simulink model "SVMInverter"  (R2022b)
settings: Solver=ode4  StartTime=0.0  StopTime=0.06  FixedStep=1e-6  RelTol=1e-3
values from neighbouring files (symbols this model uses):
  Cf = 1/(Lf*wc^2)    (= 0.000101321183642)    [FOCinit.m]
  E = 700    [FOCinit.m]
  Lf = 1e-3    (= 0.001)    [FOCinit.m]
  Ls = 0.280    (= 0.28)    [FOCinit.m]
  Poff = [1 1 1 1 1 1 1 1 1 1 1 1 1 1 1 1 1 1 ; 1 0 0 1 1 0 0 1 0 0 1 1 0 0 1 1 0 1; 1 1 0 0 1 0 0 1 1 0 0 1 1 0 1 1 0 0]'    [FOCinit.m]
  Rf = (1/(2*eps))*sqrt(Lf/Cf)    [FOCinit.m]
  Ts = 1/fs    (= 0.0001)    [FOCinit.m]
libraries: simulink_extras x6, simulink x2, mcbcontrolslib x2
settings Model: Creator=ZinouAb  LastModifiedBy=ZinouAb

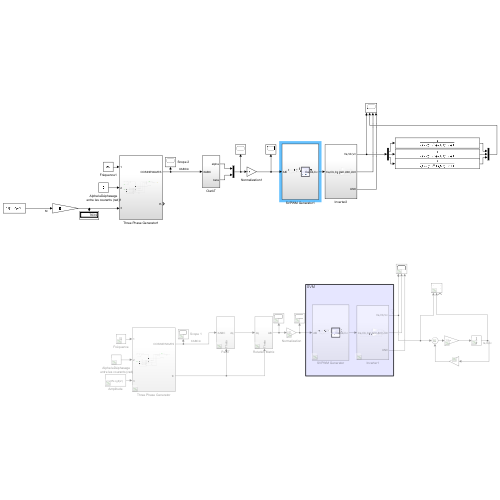
[thumbnail: Simulink's stored preview of the top-level diagram]
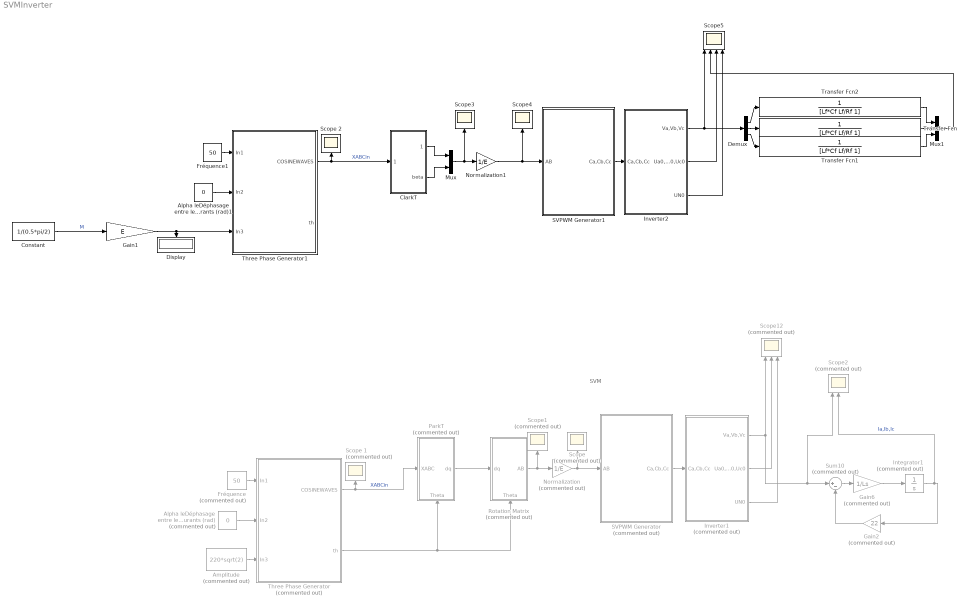
== system SVMInverter ==
  note: SVM
  Alpha leDéphasage entre les courants (rad) : Constant  Commented=on  Value=0
  Alpha leDéphasage entre les courants (rad)1 : Constant  Value=0
  Amplitude : Constant  Commented=on  Value=220*sqrt(2)
  ClarkT : Subsystem
  Constant : Constant  Value=1/(0.5*pi/2)
  Demux : Demux  Outputs=3
  Display : Display
  Fréquence : Constant  Commented=on  Value=50
  Fréquence1 : Constant  Value=50
  Gain1 : Gain  Gain=E
  Gain2 : Gain  Commented=on  Gain=22
  Gain6 : Gain  Commented=on  Gain=1/Ls
  Integrator1 : Integrator  Commented=on
  Inverter1 : Subsystem  Commented=on
  Inverter2 : Subsystem
  Mux : Mux  Inputs=2
  Mux1 : Mux  Inputs=3
  Normalization : Gain  Commented=on  Gain=1/E
  Normalization1 : Gain  Gain=1/E
  ParkT : Subsystem  Commented=on
      settings: PortSchema="{\"entries\":[{\"content\":{\"sides\":[{\"content\":{\"connectorIds\":[\"In1\"]},\"type\":\"ConnectorPlacement.EquallySpacedRectSide\",\"uuid\":\"228dfcfc-5d6b-4d2b-a954-ee5f3fee8856\"},{\"content\":{\"connectorIds\":[\"Out1\"],\"side\":\"RIGHT\"},\"type\":\"ConnectorPlacement.EquallySpacedRectSide\",\"uuid\":\"1b1b4c30-bceb-4aa5-9a3a-183aa9b64903\"},{\"content\":{\"connectorIds\":[],\"side\":\"TOP\"},\"type\":\"ConnectorPlacement.EquallySpacedRectSide\",\"uuid\":\"f7d3bddd-1df8-4cd8-ab8f-9e5cd0980ffa\"},{\"content\":{\"connectorIds\":[\"In2\"],\"side\":\"BOTTOM\"},\"type\":\"ConnectorPlacement.EquallySpacedRectSide\",\"uuid\":\"ca51e6a4-16df-4fde-8b7d-f74278a3171d\"}]},\"type\":\"ConnectorPlacement.EquallySpacedConnector\",\"uuid\":\"a8efb2f9-24b2-4419-8f97-2809a6aaa24c\"}],\"packageUris\":[\"http://schema.mathworks.com/mf0/Connector/R2020b\"],\"version\":\"1.0\"}"
  Rotation Matrix : Subsystem  Commented=on
      settings: PortSchema="{\"entries\":[{\"content\":{\"sides\":[{\"content\":{\"connectorIds\":[\"In1\"]},\"type\":\"ConnectorPlacement.EquallySpacedRectSide\",\"uuid\":\"228dfcfc-5d6b-4d2b-a954-ee5f3fee8856\"},{\"content\":{\"connectorIds\":[\"Out1\"],\"side\":\"RIGHT\"},\"type\":\"ConnectorPlacement.EquallySpacedRectSide\",\"uuid\":\"1b1b4c30-bceb-4aa5-9a3a-183aa9b64903\"},{\"content\":{\"connectorIds\":[],\"side\":\"TOP\"},\"type\":\"ConnectorPlacement.EquallySpacedRectSide\",\"uuid\":\"f7d3bddd-1df8-4cd8-ab8f-9e5cd0980ffa\"},{\"content\":{\"connectorIds\":[\"In2\"],\"side\":\"BOTTOM\"},\"type\":\"ConnectorPlacement.EquallySpacedRectSide\",\"uuid\":\"ca51e6a4-16df-4fde-8b7d-f74278a3171d\"}]},\"type\":\"ConnectorPlacement.EquallySpacedConnector\",\"uuid\":\"a8efb2f9-24b2-4419-8f97-2809a6aaa24c\"}],\"packageUris\":[\"http://schema.mathworks.com/mf0/Connector/R2020b\"],\"version\":\"1.0\"}"
  SVPWM Generator : Subsystem  Commented=on
  SVPWM Generator1 : Subsystem
  Scope : Scope  Commented=on
  Scope 1 : Scope  Commented=on
  Scope 2 : Scope
  Scope1 : Scope  Commented=on
  Scope12 : Scope  Commented=on  NumInputPorts=3
  Scope2 : Scope  Commented=on  NumInputPorts=3
  Scope3 : Scope
  Scope4 : Scope
  Scope5 : Scope  NumInputPorts=4
  Sum10 : Sum  Commented=on  Inputs=|+-
  Three Phase Generator : Subsystem  Commented=on
  Three Phase Generator1 : Subsystem
  Transfer Fcn : TransferFcn  Denominator=[Lf*Cf Lf/Rf 1]
  Transfer Fcn1 : TransferFcn  Denominator=[Lf*Cf Lf/Rf 1]
  Transfer Fcn2 : TransferFcn  Denominator=[Lf*Cf Lf/Rf 1]
  wires:
  Integrator1/1 -> Scope2/2, Gain2/1  "Ia,Ib,Ic"
  Inverter1/1(Va,Vb,Vc) -> Scope12/1, Scope2/1, Sum10/1
  Three Phase Generator/1(COSINEWAVES) -> ParkT/1(XABC), Scope 1/1  "XABCin"
  Amplitude/1 -> Three Phase Generator/3(In3)
  Alpha leDéphasage entre les courants (rad)/1 -> Three Phase Generator/2(In2)
  Fréquence/1 -> Three Phase Generator/1(In1)
  Gain2/1 -> Sum10/2
  Gain6/1 -> Integrator1/1
  Sum10/1 -> Gain6/1
  Inverter1/2(Ua0,Ub0,Uc0) -> Scope12/2
  Inverter1/3(UN0) -> Scope12/3
  Rotation Matrix/1(AB) -> Scope1/1, Normalization/1
  Normalization/1 -> SVPWM Generator/1(AB), Scope/1
  Three Phase Generator/2(th) -> ParkT/2(Theta), Rotation Matrix/2(Theta)
  ParkT/1(dq) -> Rotation Matrix/1(dq)
  SVPWM Generator/1(Ca,Cb,Cc) -> Inverter1/1(Ca,Cb,Cc)
  Three Phase Generator1/1(COSINEWAVES) -> ClarkT/1(XABC), Scope 2/1  "XABCin"
  Fréquence1/1 -> Three Phase Generator1/1(In1)
  Alpha leDéphasage entre les courants (rad)1/1 -> Three Phase Generator1/2(In2)
  ClarkT/1(alpha) -> Mux/1
  ClarkT/2(beta) -> Mux/2
  Mux/1 -> Scope3/1, Normalization1/1
  Normalization1/1 -> Scope4/1, SVPWM Generator1/1(AB)
  Inverter2/2(Ua0,Ub0,Uc0) -> Scope5/3
  Inverter2/1(Va,Vb,Vc) -> Scope5/1, Demux/1
  Inverter2/3(UN0) -> Scope5/4
  SVPWM Generator1/1(Ca,Cb,Cc) -> Inverter2/1(Ca,Cb,Cc)
  Mux1/1 -> Scope5/2
  Demux/2 -> Transfer Fcn/1
  Demux/1 -> Transfer Fcn2/1
  Demux/3 -> Transfer Fcn1/1
  Transfer Fcn/1 -> Mux1/2
  Transfer Fcn2/1 -> Mux1/1
  Transfer Fcn1/1 -> Mux1/3
  Constant/1 -> Gain1/1  "M"
  Gain1/1 -> Three Phase Generator1/3(In3), Display/1

== system SVMInverter/ClarkT ==
  XABC : Inport
  MATLAB Function1 : MATLAB Function  TreatAsAtomicUnit=on
  alpha : Outport
  beta : Outport  Port=2
  wires:
  MATLAB Function1/1(alpha) -> alpha/1
  XABC/1 -> MATLAB Function1/1(x)
  MATLAB Function1/2(beta) -> beta/1

== system SVMInverter/Inverter1 ==
  Ca,Cb,Cc : Inport
  Constant1 : Constant  Value=E
  Gain : Gain  Gain=1/3
  Gain1 : Gain  Gain=eye(3)  Multiplication=Matrix(K*u)
  Gain2 : Gain  Gain=[2 -1 -1; -1 2 -1; -1 -1 2]  Multiplication=Matrix(K*u)
  Gain6 : Gain  Gain=1/3
  Product1 : Product
  Product3 : Product
  Scope6 : Scope
  Sum of Elements : Sum  Inputs=+
  Va,Vb,Vc : Outport
  Ua0,Ub0,Uc0 : Outport  Port=2
  UN0 : Outport  Port=3
  wires:
  Gain2/1 -> Gain6/1
  Product3/1 -> Va,Vb,Vc/1  "Va,Vb,Vc"
  Ca,Cb,Cc/1 -> Gain1/1, [Cmd], Gain2/1, Scope6/1  "Ca,Cb,Cc"
  Constant1/1 -> Product1/2, Product3/2  "U0"
  Gain6/1 -> Product3/1
  Gain1/1 -> Product1/1
  Product1/1 -> Sum of Elements/1, Ua0,Ub0,Uc0/1  "Ua0,Ub0,Uc0"
  Sum of Elements/1 -> Gain/1
  Gain/1 -> UN0/1

== system SVMInverter/Inverter2 ==
  Ca,Cb,Cc : Inport
  Constant1 : Constant  Value=E
  Gain : Gain  Gain=1/3
  Gain1 : Gain  Gain=eye(3)  Multiplication=Matrix(K*u)
  Gain2 : Gain  Gain=[2 -1 -1; -1 2 -1; -1 -1 2]  Multiplication=Matrix(K*u)
  Gain6 : Gain  Gain=1/3
  Product1 : Product
  Product3 : Product
  Scope6 : Scope
  Sum of Elements : Sum  Inputs=+
  Va,Vb,Vc : Outport
  Ua0,Ub0,Uc0 : Outport  Port=2
  UN0 : Outport  Port=3
  wires:
  Gain2/1 -> Gain6/1
  Product3/1 -> Va,Vb,Vc/1  "Va,Vb,Vc"
  Ca,Cb,Cc/1 -> Gain1/1, [Cmd], Gain2/1, Scope6/1  "Ca,Cb,Cc"
  Constant1/1 -> Product1/2, Product3/2  "U0"
  Gain6/1 -> Product3/1
  Gain1/1 -> Product1/1
  Product1/1 -> Sum of Elements/1, Ua0,Ub0,Uc0/1  "Ua0,Ub0,Uc0"
  Sum of Elements/1 -> Gain/1
  Gain/1 -> UN0/1

== system SVMInverter/ParkT ==
  XABC : Inport
  Theta : Inport  Port=2
  MATLAB Function1 : MATLAB Function  TreatAsAtomicUnit=on
  dq : Outport
  wires:
  Theta/1 -> MATLAB Function1/2(th)
  MATLAB Function1/1(dq) -> dq/1
  XABC/1 -> MATLAB Function1/1(x)

== system SVMInverter/Rotation Matrix ==
  dq : Inport
  Theta : Inport  Port=2
  MATLAB Function1 : MATLAB Function  TreatAsAtomicUnit=on
  AB : Outport
  wires:
  Theta/1 -> MATLAB Function1/2(th)
  MATLAB Function1/1(AB) -> AB/1
  dq/1 -> MATLAB Function1/1(x)

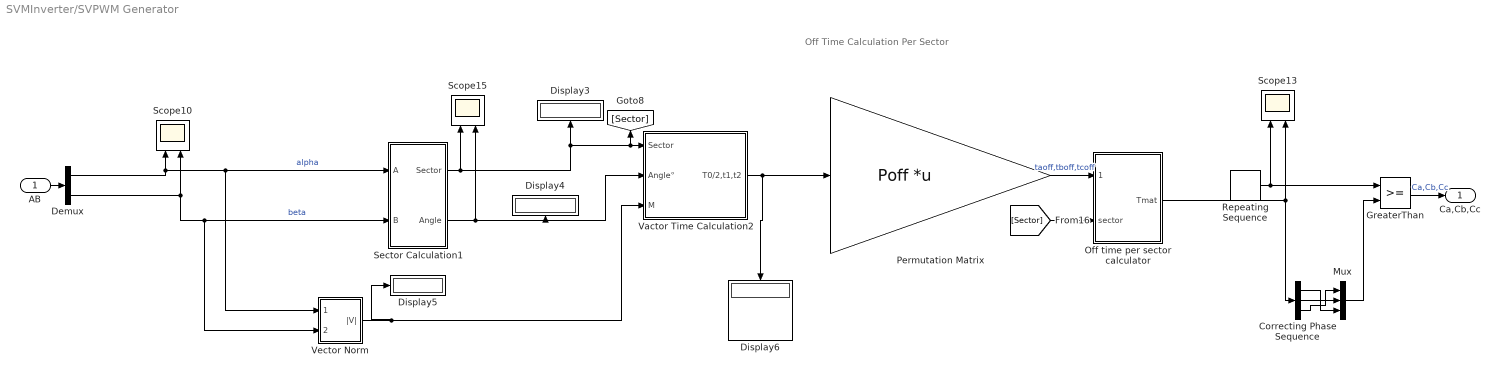
== system SVMInverter/SVPWM Generator ==
  note: Off Time Calculation Per Sector
  AB : Inport
  Correcting Phase Sequence : Demux  Outputs=3
  Demux : Demux  Outputs=2
  Display{3..6} (4 alike) : Display
  GreaterThan : RelationalOperator  OutDataTypeStr=boolean  RndMeth=Simplest  InputSameDT=off
  Mux : Mux  Inputs=3
  Off time per sector calculator : Subsystem
  Permutation Matrix : Gain  Gain=Poff  Multiplication=Matrix(K*u)
  Repeating Sequence : simulink/Sources/Repeating Sequence  rep_seq_t=[0 Ts 2*Ts]  rep_seq_y=[0 1 0]
  Scope10 : Scope  NumInputPorts=2
  Scope13 : Scope  NumInputPorts=2
  Scope15 : Scope  NumInputPorts=2
  Sector Calculation1 : Subsystem
  Vactor Time Calculation2 : Subsystem
  Vector Norm : Subsystem
  Ca,Cb,Cc : Outport
  wires:
  Demux/2 -> Vector Norm/2(Beta), Sector Calculation1/2(B), Scope10/2  "beta"
  Sector Calculation1/1(Sector) -> Scope15/1, Vactor Time Calculation2/1(Sector), [Sector], Display3/1
  Off time per sector calculator/1(Tmat) -> Correcting Phase Sequence/1, Scope13/2
  [Sector] -> Off time per sector calculator/2(sector)
  Demux/1 -> Scope10/1, Vector Norm/1(alpha), Sector Calculation1/1(A)  "alpha"
  Repeating Sequence/1 -> Scope13/1, GreaterThan/1
  Sector Calculation1/2(Angle) -> Vactor Time Calculation2/2(Angle°), Display4/1, Scope15/2
  Vactor Time Calculation2/1(T0/2,t1,t2) -> Permutation Matrix/1, Display6/1
  Permutation Matrix/1 -> Off time per sector calculator/1(taoff,tboff,tcoff)  "taoff,tboff,tcoff"
  Vector Norm/1(|V|) -> Vactor Time Calculation2/3(M), Display5/1
  GreaterThan/1 -> Ca,Cb,Cc/1  "Ca,Cb,Cc"
  AB/1 -> Demux/1
  Correcting Phase Sequence/1 -> Mux/3
  Correcting Phase Sequence/3 -> Mux/1
  Correcting Phase Sequence/2 -> Mux/2
  Mux/1 -> GreaterThan/2

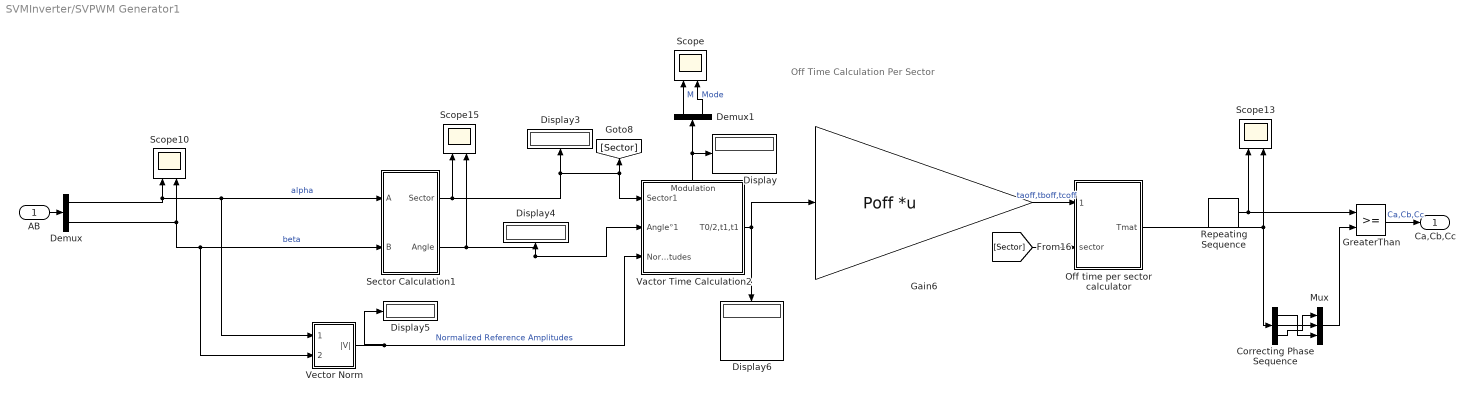
== system SVMInverter/SVPWM Generator1 ==
  note: Off Time Calculation Per Sector
  AB : Inport
  Correcting Phase Sequence : Demux  Outputs=3
  Demux : Demux  Outputs=2
  Demux1 : Demux  Outputs=2
  Display{,3..6} (5 alike) : Display
  Gain6 : Gain  Gain=Poff  Multiplication=Matrix(K*u)
  GreaterThan : RelationalOperator  OutDataTypeStr=boolean  RndMeth=Simplest  InputSameDT=off
  Mux : Mux  Inputs=3
  Off time per sector calculator : Subsystem
  Repeating Sequence : simulink/Sources/Repeating Sequence  rep_seq_t=[0 Ts 2*Ts]  rep_seq_y=[0 1 0]
  Scope{,10,13,15} (4 alike) : Scope  NumInputPorts=2
  Sector Calculation1 : Subsystem
  Vactor Time Calculation2 : Subsystem
      settings: PortSchema="{\"entries\":[{\"content\":{\"sides\":[{\"content\":{\"connectorIds\":[\"In1\",\"In2\",\"In3\"]},\"type\":\"ConnectorPlacement.EquallySpacedRectSide\",\"uuid\":\"b36ff3f1-d1b6-4cc1-9bbd-425fd19c1a38\"},{\"content\":{\"connectorIds\":[\"Out1\"],\"side\":\"RIGHT\"},\"type\":\"ConnectorPlacement.EquallySpacedRectSide\",\"uuid\":\"a221f04d-f18a-44c3-93a1-83af2c15186c\"},{\"content\":{\"connectorIds\":[\"Out2\"],\"side\":\"TOP\"},\"type\":\"ConnectorPlacement.EquallySpacedRectSide\",\"uuid\":\"f879d1f5-8adc-45c1-bee9-dc1dc3f910d6\"}]},\"type\":\"ConnectorPlacement.EquallySpacedConnector\",\"uuid\":\"747b21c6-a5ea-4368-bf31-a8fc38ff0719\"}],\"packageUris\":[\"http://schema.mathworks.com/mf0/Connector/R2020b\"],\"version\":\"1.0\"}"
  Vector Norm : Subsystem
  Ca,Cb,Cc : Outport
  wires:
  Demux/2 -> Vector Norm/2(Beta), Sector Calculation1/2(B), Scope10/2  "beta"
  Sector Calculation1/1(Sector) -> Scope15/1, Vactor Time Calculation2/1(Sector1), [Sector], Display3/1
  Off time per sector calculator/1(Tmat) -> Correcting Phase Sequence/1, Scope13/2
  [Sector] -> Off time per sector calculator/2(sector)
  Demux/1 -> Scope10/1, Vector Norm/1(alpha), Sector Calculation1/1(A)  "alpha"
  Repeating Sequence/1 -> Scope13/1, GreaterThan/1
  Sector Calculation1/2(Angle) -> Vactor Time Calculation2/2(Angle°1), Display4/1, Scope15/2
  Gain6/1 -> Off time per sector calculator/1(taoff,tboff,tcoff)  "taoff,tboff,tcoff"
  GreaterThan/1 -> Ca,Cb,Cc/1  "Ca,Cb,Cc"
  AB/1 -> Demux/1
  Correcting Phase Sequence/1 -> Mux/3
  Correcting Phase Sequence/3 -> Mux/1
  Correcting Phase Sequence/2 -> Mux/2
  Mux/1 -> GreaterThan/2
  Vector Norm/1(|V|) -> Vactor Time Calculation2/3(Normalized Reference Amplitudes), Display5/1  "Normalized Reference Amplitudes"
  Vactor Time Calculation2/1(T0/2,t1,t1) -> Gain6/1, Display6/1
  Vactor Time Calculation2/2(Modulation) -> Demux1/1, Display/1
  Demux1/1 -> Scope/1  "M"
  Demux1/2 -> Scope/2  "Mode"

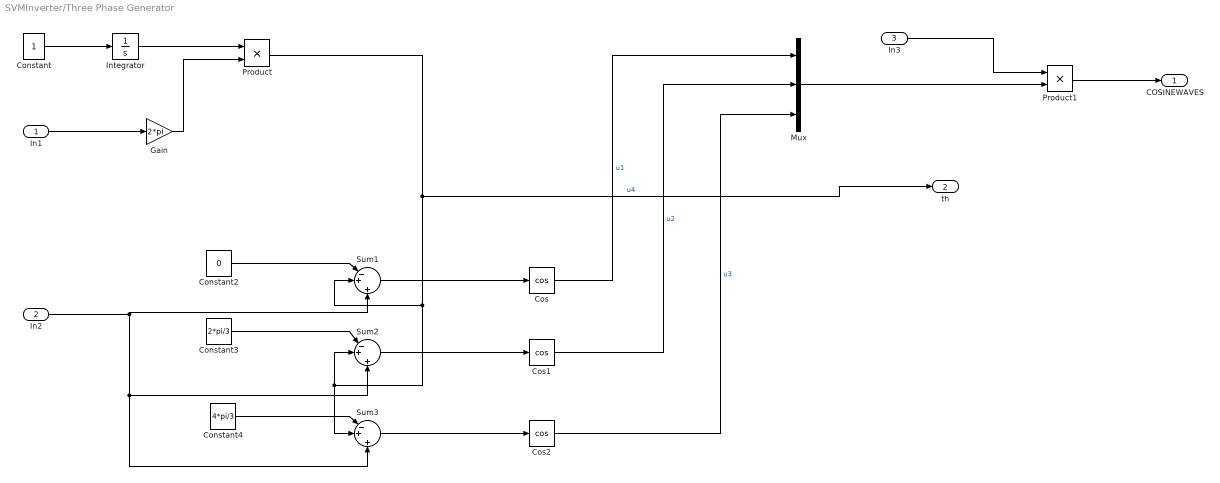
== system SVMInverter/Three Phase Generator ==
  In1 : Inport
  In2 : Inport  Port=2
  In3 : Inport  Port=3
  Constant : Constant
  Constant2 : Constant  Value=0
  Constant3 : Constant  Value=2*pi/3
  Constant4 : Constant  Value=4*pi/3
  Cos : Trigonometry  Operator=cos
  Cos1 : Trigonometry  Operator=cos
  Cos2 : Trigonometry  Operator=cos
  Gain : Gain  Gain=2*pi
  Integrator : Integrator
  Mux : Mux  Inputs=3
  Product : Product
  Product1 : Product
  Sum1 : Sum  Inputs=|-+|+
  Sum2 : Sum  Inputs=|-+|+
  Sum3 : Sum  Inputs=|-+|+
  COSINEWAVES : Outport
  th : Outport  Port=2
  wires:
  Constant/1 -> Integrator/1
  Sum2/1 -> Cos1/1
  In2/1 -> Sum1/3, Sum3/3, Sum2/3
  Product/1 -> th/1, Sum3/2, Sum2/2, Sum1/2  "u4"
  Constant3/1 -> Sum2/1
  Sum3/1 -> Cos2/1
  Sum1/1 -> Cos/1
  Constant2/1 -> Sum1/1
  Constant4/1 -> Sum3/1
  Gain/1 -> Product/2
  Integrator/1 -> Product/1
  In1/1 -> Gain/1
  Cos1/1 -> Mux/2  "u2"
  Cos/1 -> Mux/1  "u1"
  Cos2/1 -> Mux/3  "u3"
  Mux/1 -> Product1/2
  In3/1 -> Product1/1
  Product1/1 -> COSINEWAVES/1

== system SVMInverter/Three Phase Generator1 ==
  In1 : Inport
  In2 : Inport  Port=2
  In3 : Inport  Port=3
  Constant : Constant
  Constant2 : Constant  Value=0
  Constant3 : Constant  Value=2*pi/3
  Constant4 : Constant  Value=4*pi/3
  Cos : Trigonometry  Operator=cos
  Cos1 : Trigonometry  Operator=cos
  Cos2 : Trigonometry  Operator=cos
  Gain : Gain  Gain=2*pi
  Integrator : Integrator
  Mux : Mux  Inputs=3
  Product : Product
  Product1 : Product
  Sum1 : Sum  Inputs=|-+|+
  Sum2 : Sum  Inputs=|-+|+
  Sum3 : Sum  Inputs=|-+|+
  COSINEWAVES : Outport
  th : Outport  Port=2
  wires:
  Constant/1 -> Integrator/1
  Sum2/1 -> Cos1/1
  In2/1 -> Sum1/3, Sum3/3, Sum2/3
  Product/1 -> th/1, Sum3/2, Sum2/2, Sum1/2  "u4"
  Constant3/1 -> Sum2/1
  Sum3/1 -> Cos2/1
  Sum1/1 -> Cos/1
  Constant2/1 -> Sum1/1
  Constant4/1 -> Sum3/1
  Gain/1 -> Product/2
  Integrator/1 -> Product/1
  In1/1 -> Gain/1
  Cos1/1 -> Mux/2  "u2"
  Cos/1 -> Mux/1  "u1"
  Cos2/1 -> Mux/3  "u3"
  Mux/1 -> Product1/2
  In3/1 -> Product1/1
  Product1/1 -> COSINEWAVES/1

== system SVMInverter/SVPWM Generator/Off time per sector calculator ==
  taoff,tboff,tcoff : Inport
  sector : Inport  Port=2
  Off time per sector calculator : MATLAB Function  TreatAsAtomicUnit=on
  Tmat : Outport
  wires:
  Off time per sector calculator/1(Tmat) -> Tmat/1
  sector/1 -> Off time per sector calculator/2(sector)
  taoff,tboff,tcoff/1 -> Off time per sector calculator/1(toff)

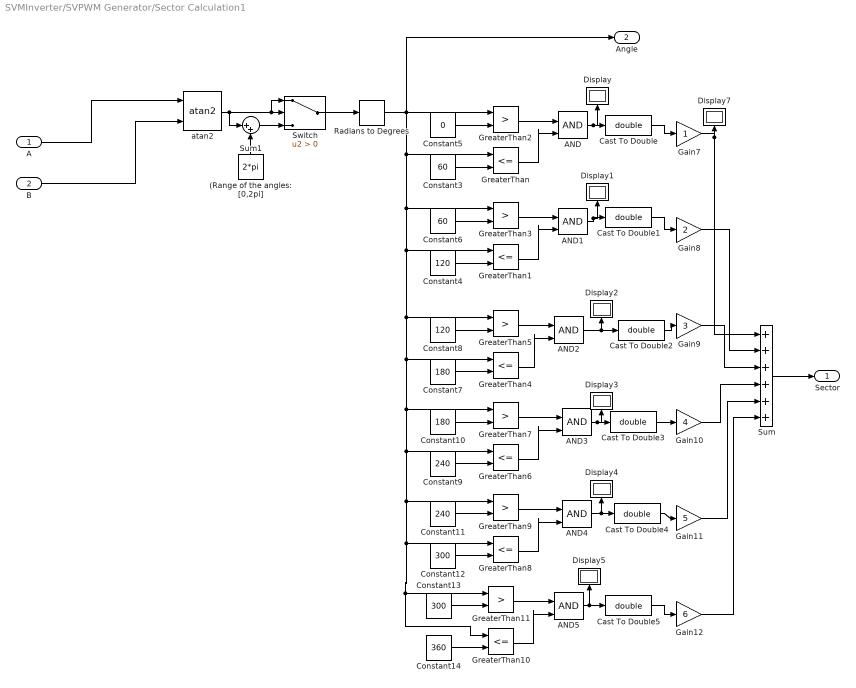
== system SVMInverter/SVPWM Generator/Sector Calculation1 ==
  A : Inport
  B : Inport  Port=2
  (Range of the angles: [0,2pi] : Constant  Value=2*pi
  AND{,1..5} (6 alike) : Logic  IconShape=distinctive  AllPortsSameDT=off  OutDataTypeStr=boolean
  Cast To Double{,1..5} (6 alike) : DataTypeConversion  OutDataTypeStr=double  SaturateOnIntegerOverflow=off  RndMeth=Floor
  Constant10 : Constant  Value=180
  Constant11 : Constant  Value=240
  Constant12 : Constant  Value=300
  Constant13 : Constant  Value=300
  Constant14 : Constant  Value=360
  Constant3 : Constant  Value=60
  Constant4 : Constant  Value=120
  Constant5 : Constant  Value=0
  Constant6 : Constant  Value=60
  Constant7 : Constant  Value=180
  Constant8 : Constant  Value=120
  Constant9 : Constant  Value=240
  Display{,1..5,7} (7 alike) : Display
  Gain10 : Gain  Gain=4
  Gain11 : Gain  Gain=5
  Gain12 : Gain  Gain=6
  Gain7 : Gain
  Gain8 : Gain  Gain=2
  Gain9 : Gain  Gain=3
  GreaterThan{,1,4,6,8,10} (6 alike) : RelationalOperator  Operator=<=  OutDataTypeStr=boolean  RndMeth=Simplest  InputSameDT=off
  GreaterThan{2..3,5,7,9,11} (6 alike) : RelationalOperator  Operator=>  OutDataTypeStr=boolean  RndMeth=Simplest  InputSameDT=off
  Radians to Degrees : simulink_extras/Transformations/Radians to Degrees
  Sum : Sum  Inputs=++++++
  Sum1 : Sum  Inputs=|++
  Switch : Switch  Criteria=u2 > Threshold  SaturateOnIntegerOverflow=off  InputSameDT=off
  atan2 : mcbcontrolslib/atan2  outputUnit=Radians
      settings: LibrarySourceBlock=mcblib/Controls/Math Transforms/atan2
  Sector : Outport
  Angle : Outport  Port=2
  wires:
  AND3/1 -> Cast To Double3/1, Display3/1
  Sum/1 -> Sector/1
  B/1 -> atan2/2
  A/1 -> atan2/1
  Cast To Double1/1 -> Gain8/1
  Cast To Double5/1 -> Gain12/1
  Constant6/1 -> GreaterThan3/2
  Gain7/1 -> Display7/1, Sum/1
  GreaterThan7/1 -> AND3/1
  Cast To Double2/1 -> Gain9/1
  Constant3/1 -> GreaterThan/2
  Cast To Double3/1 -> Gain10/1
  GreaterThan2/1 -> AND/1
  Constant9/1 -> GreaterThan6/2
  Cast To Double/1 -> Gain7/1
  GreaterThan11/1 -> AND5/1
  Gain10/1 -> Sum/4
  Gain11/1 -> Sum/5
  GreaterThan9/1 -> AND4/1
  Cast To Double4/1 -> Gain11/1
  Constant11/1 -> GreaterThan9/2
  Constant5/1 -> GreaterThan2/2
  Constant12/1 -> GreaterThan8/2
  Constant10/1 -> GreaterThan7/2
  Constant7/1 -> GreaterThan4/2
  AND4/1 -> Cast To Double4/1, Display4/1
  AND/1 -> Cast To Double/1, Display/1
  AND5/1 -> Cast To Double5/1, Display5/1
  Constant8/1 -> GreaterThan5/2
  GreaterThan6/1 -> AND3/2
  GreaterThan/1 -> AND/2
  Gain9/1 -> Sum/3
  AND2/1 -> Cast To Double2/1, Display2/1
  GreaterThan4/1 -> AND2/2
  Gain12/1 -> Sum/6
  Constant13/1 -> GreaterThan11/2
  Gain8/1 -> Sum/2
  GreaterThan8/1 -> AND4/2
  GreaterThan1/1 -> AND1/2
  Constant14/1 -> GreaterThan10/2
  GreaterThan3/1 -> AND1/1
  Constant4/1 -> GreaterThan1/2
  Radians to Degrees/1 -> GreaterThan2/1, GreaterThan/1, GreaterThan3/1, GreaterThan1/1, GreaterThan5/1, GreaterThan4/1, GreaterThan7/1, GreaterThan6/1, GreaterThan9/1, GreaterThan8/1, GreaterThan11/1, GreaterThan10/1, Angle/1
  GreaterThan10/1 -> AND5/2
  GreaterThan5/1 -> AND2/1
  AND1/1 -> Cast To Double1/1, Display1/1
  (Range of the angles: [0,2pi]/1 -> Sum1/2
  atan2/1 -> Sum1/1, Switch/1, Switch/2
  Sum1/1 -> Switch/3
  Switch/1 -> Radians to Degrees/1

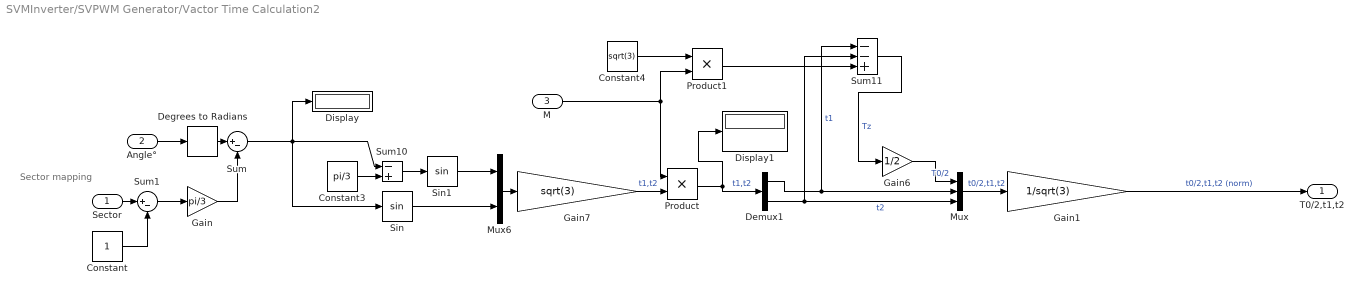
== system SVMInverter/SVPWM Generator/Vactor Time Calculation2 ==
  note: Sector mapping
  Sector : Inport
  Angle° : Inport  Port=2
  M : Inport  Port=3
  Constant : Constant
  Constant3 : Constant  Value=pi/3
  Constant4 : Constant  Value=sqrt(3)
  Degrees to Radians : simulink_extras/Transformations/Degrees to Radians
  Demux1 : Demux  Outputs=2
  Display : Display
  Display1 : Display
  Gain : Gain  Gain=pi/3
  Gain1 : Gain  Gain=1/sqrt(3)
  Gain6 : Gain  Gain=1/2
  Gain7 : Gain  Gain=sqrt(3)
  Mux : Mux  Inputs=3
  Mux6 : Mux  Inputs=2
  Product : Product
  Product1 : Product
  Sin : Trigonometry
  Sin1 : Trigonometry
  Sum : Sum  Inputs=|+-
  Sum1 : Sum  Inputs=|+-
  Sum10 : Sum  Inputs=-+
  Sum11 : Sum  Inputs=--+
  T0/2,t1,t2 : Outport
  wires:
  Product1/1 -> Sum11/3
  Sum11/1 -> Gain6/1  "Tz"
  Demux1/1 -> Mux/2, Sum11/1  "t1"
  Demux1/2 -> Mux/3, Sum11/2  "t2"
  Mux6/1 -> Gain7/1
  Product/1 -> Demux1/1, Display1/1  "t1,t2"
  Gain6/1 -> Mux/1  "T0/2"
  Angle°/1 -> Degrees to Radians/1
  Sin/1 -> Mux6/2
  Sin1/1 -> Mux6/1
  Constant3/1 -> Sum10/2
  Sum10/1 -> Sin1/1
  Sum/1 -> Sin/1, Display/1, Sum10/1
  Gain7/1 -> Product/2  "t1,t2"
  Mux/1 -> Gain1/1  "t0/2,t1,t2"
  Gain1/1 -> T0/2,t1,t2/1  "t0/2,t1,t2 (norm)"
  Degrees to Radians/1 -> Sum/1
  Gain/1 -> Sum/2
  Sector/1 -> Sum1/1
  Constant/1 -> Sum1/2
  Sum1/1 -> Gain/1
  Constant4/1 -> Product1/1
  M/1 -> Product1/2, Product/1

== system SVMInverter/SVPWM Generator/Vector Norm ==
  alpha : Inport
  Beta : Inport  Port=2
  Square : Math  Operator=square
  Square Root : Sqrt
  Square1 : Math  Operator=square
  Sum13 : Sum  Inputs=|++
  |V| : Outport
  wires:
  Square/1 -> Sum13/2
  Square1/1 -> Sum13/1
  Beta/1 -> Square/1
  Square Root/1 -> |V|/1
  Sum13/1 -> Square Root/1
  alpha/1 -> Square1/1

== system SVMInverter/SVPWM Generator1/Off time per sector calculator ==
  taoff,tboff,tcoff : Inport
  sector : Inport  Port=2
  Off time per sector calculator : MATLAB Function  TreatAsAtomicUnit=on
  Tmat : Outport
  wires:
  Off time per sector calculator/1(Tmat) -> Tmat/1
  sector/1 -> Off time per sector calculator/2(sector)
  taoff,tboff,tcoff/1 -> Off time per sector calculator/1(toff)

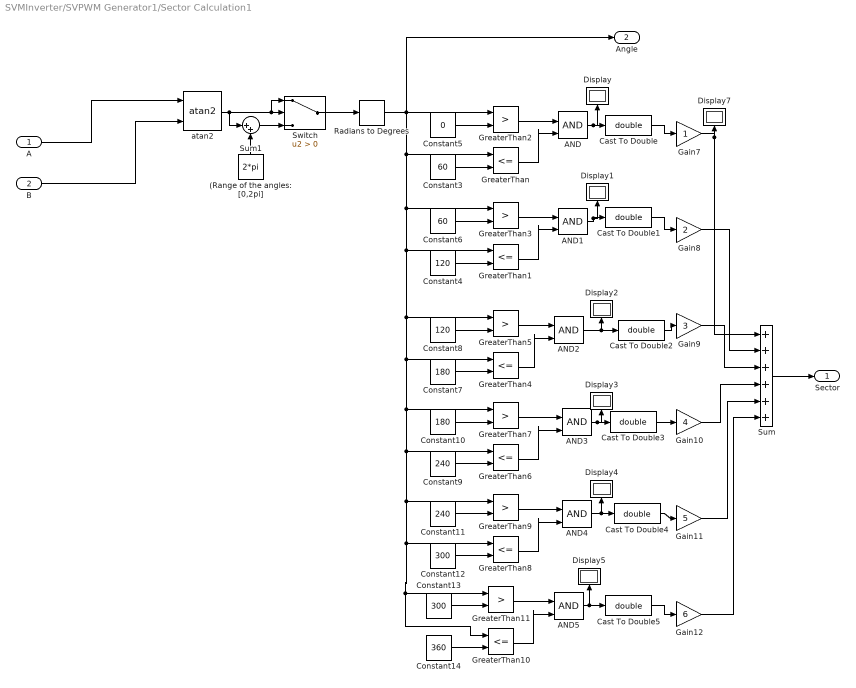
== system SVMInverter/SVPWM Generator1/Sector Calculation1 ==
  A : Inport
  B : Inport  Port=2
  (Range of the angles: [0,2pi] : Constant  Value=2*pi
  AND{,1..5} (6 alike) : Logic  IconShape=distinctive  AllPortsSameDT=off  OutDataTypeStr=boolean
  Cast To Double{,1..5} (6 alike) : DataTypeConversion  OutDataTypeStr=double  SaturateOnIntegerOverflow=off  RndMeth=Floor
  Constant10 : Constant  Value=180
  Constant11 : Constant  Value=240
  Constant12 : Constant  Value=300
  Constant13 : Constant  Value=300
  Constant14 : Constant  Value=360
  Constant3 : Constant  Value=60
  Constant4 : Constant  Value=120
  Constant5 : Constant  Value=0
  Constant6 : Constant  Value=60
  Constant7 : Constant  Value=180
  Constant8 : Constant  Value=120
  Constant9 : Constant  Value=240
  Display{,1..5,7} (7 alike) : Display
  Gain10 : Gain  Gain=4
  Gain11 : Gain  Gain=5
  Gain12 : Gain  Gain=6
  Gain7 : Gain
  Gain8 : Gain  Gain=2
  Gain9 : Gain  Gain=3
  GreaterThan{,1,4,6,8,10} (6 alike) : RelationalOperator  Operator=<=  OutDataTypeStr=boolean  RndMeth=Simplest  InputSameDT=off
  GreaterThan{2..3,5,7,9,11} (6 alike) : RelationalOperator  Operator=>  OutDataTypeStr=boolean  RndMeth=Simplest  InputSameDT=off
  Radians to Degrees : simulink_extras/Transformations/Radians to Degrees
  Sum : Sum  Inputs=++++++
  Sum1 : Sum  Inputs=|++
  Switch : Switch  Criteria=u2 > Threshold  SaturateOnIntegerOverflow=off  InputSameDT=off
  atan2 : mcbcontrolslib/atan2  outputUnit=Radians
      settings: LibrarySourceBlock=mcblib/Controls/Math Transforms/atan2
  Sector : Outport
  Angle : Outport  Port=2
  wires:
  AND3/1 -> Cast To Double3/1, Display3/1
  Sum/1 -> Sector/1
  B/1 -> atan2/2
  A/1 -> atan2/1
  Cast To Double1/1 -> Gain8/1
  Cast To Double5/1 -> Gain12/1
  Constant6/1 -> GreaterThan3/2
  Gain7/1 -> Display7/1, Sum/1
  GreaterThan7/1 -> AND3/1
  Cast To Double2/1 -> Gain9/1
  Constant3/1 -> GreaterThan/2
  Cast To Double3/1 -> Gain10/1
  GreaterThan2/1 -> AND/1
  Constant9/1 -> GreaterThan6/2
  Cast To Double/1 -> Gain7/1
  GreaterThan11/1 -> AND5/1
  Gain10/1 -> Sum/4
  Gain11/1 -> Sum/5
  GreaterThan9/1 -> AND4/1
  Cast To Double4/1 -> Gain11/1
  Constant11/1 -> GreaterThan9/2
  Constant5/1 -> GreaterThan2/2
  Constant12/1 -> GreaterThan8/2
  Constant10/1 -> GreaterThan7/2
  Constant7/1 -> GreaterThan4/2
  AND4/1 -> Cast To Double4/1, Display4/1
  AND/1 -> Cast To Double/1, Display/1
  AND5/1 -> Cast To Double5/1, Display5/1
  Constant8/1 -> GreaterThan5/2
  GreaterThan6/1 -> AND3/2
  GreaterThan/1 -> AND/2
  Gain9/1 -> Sum/3
  AND2/1 -> Cast To Double2/1, Display2/1
  GreaterThan4/1 -> AND2/2
  Gain12/1 -> Sum/6
  Constant13/1 -> GreaterThan11/2
  Gain8/1 -> Sum/2
  GreaterThan8/1 -> AND4/2
  GreaterThan1/1 -> AND1/2
  Constant14/1 -> GreaterThan10/2
  GreaterThan3/1 -> AND1/1
  Constant4/1 -> GreaterThan1/2
  Radians to Degrees/1 -> GreaterThan2/1, GreaterThan/1, GreaterThan3/1, GreaterThan1/1, GreaterThan5/1, GreaterThan4/1, GreaterThan7/1, GreaterThan6/1, GreaterThan9/1, GreaterThan8/1, GreaterThan11/1, GreaterThan10/1, Angle/1
  GreaterThan10/1 -> AND5/2
  GreaterThan5/1 -> AND2/1
  AND1/1 -> Cast To Double1/1, Display1/1
  (Range of the angles: [0,2pi]/1 -> Sum1/2
  atan2/1 -> Sum1/1, Switch/1, Switch/2
  Sum1/1 -> Switch/3
  Switch/1 -> Radians to Degrees/1

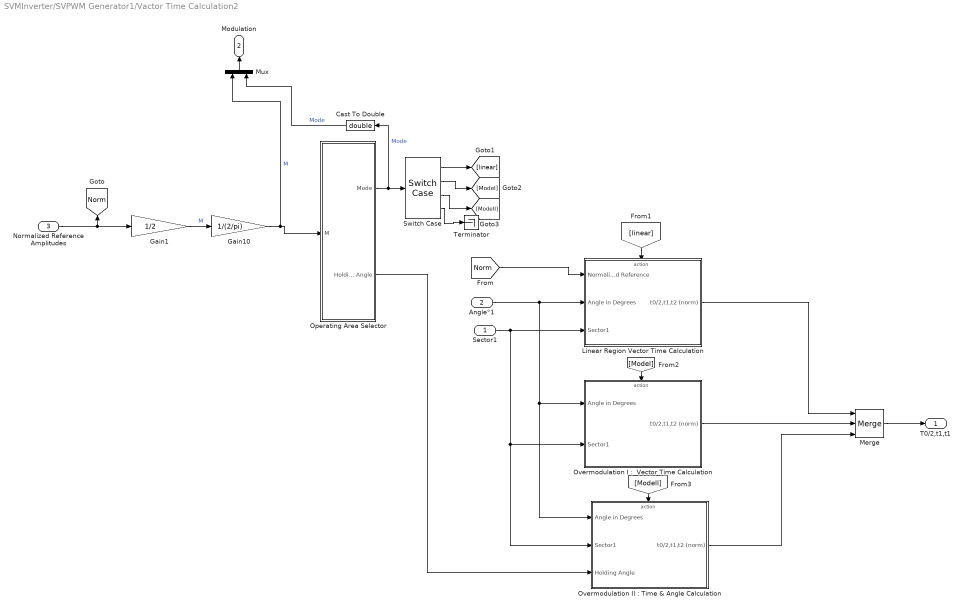
== system SVMInverter/SVPWM Generator1/Vactor Time Calculation2 ==
  Sector1 : Inport
  Angle°1 : Inport  Port=2
  Normalized Reference Amplitudes : Inport  Port=3
  Cast To Double : DataTypeConversion  OutDataTypeStr=double  SaturateOnIntegerOverflow=off  RndMeth=Floor
  Gain1 : Gain  Gain=1/2
  Gain10 : Gain  Gain=1/(2/pi)
  Linear Region Vector Time Calculation : Subsystem  TreatAsAtomicUnit=on
  Merge : Merge  Inputs=3
  Mux : Mux  Inputs=2
  Operating Area Selector : Subsystem
  "Overmodulation I :  Vector Time Calculation" : Subsystem  TreatAsAtomicUnit=on
  "Overmodulation II : Time & Angle Calculation" : Subsystem  TreatAsAtomicUnit=on
  Switch Case : SwitchCase  CaseConditions={0,1,2}
  Terminator : Terminator
  T0/2,t1,t1 : Outport
  Modulation : Outport  Port=2
  tag scope: Norm=global
  wires:
  Normalized Reference Amplitudes/1 -> Gain1/1, [Norm]
  Gain10/1 -> Operating Area Selector/1(M), Mux/1  "M"
  [Norm] -> Linear Region Vector Time Calculation/1("Normalized Reference ")
  Sector1/1 -> "Overmodulation II : Time & Angle Calculation"/2(Sector1), "Overmodulation I :  Vector Time Calculation"/2(Sector1), Linear Region Vector Time Calculation/3(Sector1)
  Merge/1 -> T0/2,t1,t1/1
  Linear Region Vector Time Calculation/1(t0/2,t1,t2 (norm)) -> Merge/1
  Operating Area Selector/2(Holding Angle) -> "Overmodulation II : Time & Angle Calculation"/3(Holding Angle)
  Switch Case/1 -> [linear]
  Switch Case/2 -> [ModeI]
  Switch Case/3 -> [ModeII]
  [linear] -> Linear Region Vector Time Calculation/Action
  Angle°1/1 -> "Overmodulation II : Time & Angle Calculation"/1("Angle in Degrees "), "Overmodulation I :  Vector Time Calculation"/1("Angle in Degrees "), Linear Region Vector Time Calculation/2("Angle in Degrees ")
  Operating Area Selector/1(Mode) -> Cast To Double/1, Switch Case/1  "Mode"
  Mux/1 -> Modulation/1
  Cast To Double/1 -> Mux/2  "Mode"
  "Overmodulation I :  Vector Time Calculation"/1(t0/2,t1,t2 (norm)) -> Merge/2
  "Overmodulation II : Time & Angle Calculation"/1(t0/2,t1,t2 (norm)) -> Merge/3
  [ModeI] -> "Overmodulation I :  Vector Time Calculation"/Action
  [ModeII] -> "Overmodulation II : Time & Angle Calculation"/Action
  Switch Case/4 -> Terminator/1
  Gain1/1 -> Gain10/1  "M"

== system SVMInverter/SVPWM Generator1/Vector Norm ==
  alpha : Inport
  Beta : Inport  Port=2
  Square : Math  Operator=square
  Square Root : Sqrt
  Square1 : Math  Operator=square
  Sum13 : Sum  Inputs=|++
  |V| : Outport
  wires:
  Square/1 -> Sum13/2
  Square1/1 -> Sum13/1
  Beta/1 -> Square/1
  Square Root/1 -> |V|/1
  Sum13/1 -> Square Root/1
  alpha/1 -> Square1/1

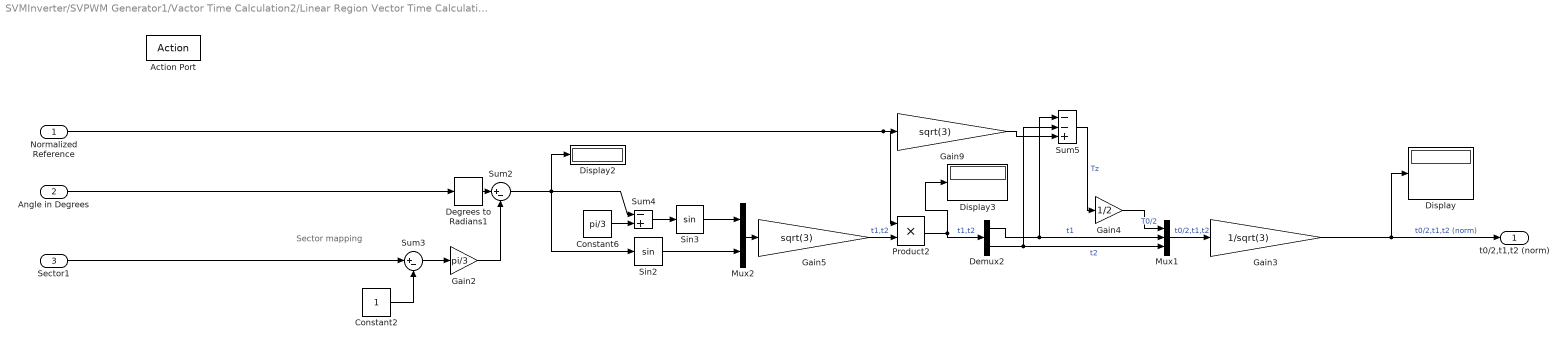
== system SVMInverter/SVPWM Generator1/Vactor Time Calculation2/Linear Region Vector Time Calculation ==
  note: Sector mapping
  "Normalized Reference " : Inport
  "Angle in Degrees " : Inport  Port=2
  Sector1 : Inport  Port=3
  Action Port : ActionPort  InitializeStates=reset  ActionPortLabel=case [ 0 ]:
  Constant2 : Constant
  Constant6 : Constant  Value=pi/3
  Degrees to Radians1 : simulink_extras/Transformations/Degrees to Radians
  Demux2 : Demux  Outputs=2
  Display : Display
  Display2 : Display
  Display3 : Display
  Gain2 : Gain  Gain=pi/3
  Gain3 : Gain  Gain=1/sqrt(3)
  Gain4 : Gain  Gain=1/2
  Gain5 : Gain  Gain=sqrt(3)
  Gain9 : Gain  Gain=sqrt(3)
  Mux1 : Mux  Inputs=3
  Mux2 : Mux  Inputs=2
  Product2 : Product
  Sin2 : Trigonometry
  Sin3 : Trigonometry
  Sum2 : Sum  Inputs=|+-
  Sum3 : Sum  Inputs=|+-
  Sum4 : Sum  Inputs=-+
  Sum5 : Sum  Inputs=--+
  t0/2,t1,t2 (norm) : Outport
  wires:
  Gain2/1 -> Sum2/2
  Gain3/1 -> Display/1, t0/2,t1,t2 (norm)/1  "t0/2,t1,t2 (norm)"
  Sum5/1 -> Gain4/1  "Tz"
  Gain4/1 -> Mux1/1  "T0/2"
  "Angle in Degrees "/1 -> Degrees to Radians1/1
  Constant2/1 -> Sum3/2
  Constant6/1 -> Sum4/2
  Gain9/1 -> Sum5/3
  Sum3/1 -> Gain2/1
  Demux2/2 -> Mux1/3, Sum5/2  "t2"
  Sin3/1 -> Mux2/1
  Gain5/1 -> Product2/2  "t1,t2"
  Sum4/1 -> Sin3/1
  Mux2/1 -> Gain5/1
  Sector1/1 -> Sum3/1
  Degrees to Radians1/1 -> Sum2/1
  Demux2/1 -> Mux1/2, Sum5/1  "t1"
  Sin2/1 -> Mux2/2
  Sum2/1 -> Sin2/1, Display2/1, Sum4/1
  Mux1/1 -> Gain3/1  "t0/2,t1,t2"
  "Normalized Reference "/1 -> Product2/1, Gain9/1
  Product2/1 -> Demux2/1, Display3/1  "t1,t2"

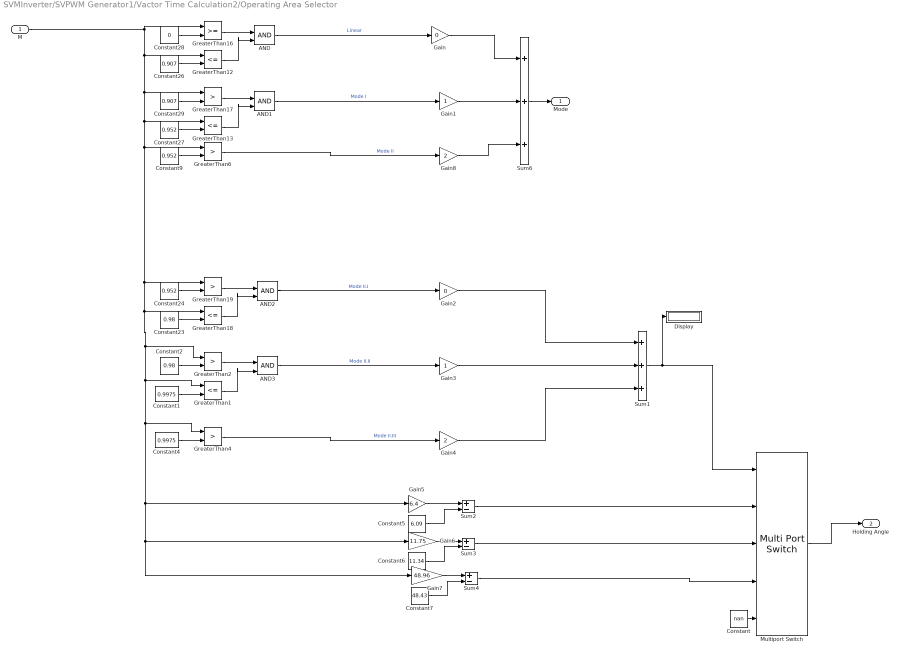
== system SVMInverter/SVPWM Generator1/Vactor Time Calculation2/Operating Area Selector ==
  M : Inport
  AND{,1..3} (4 alike) : Logic  IconShape=distinctive  AllPortsSameDT=off  OutDataTypeStr=boolean
  Constant : Constant  Value=nan
  Constant1 : Constant  Value=0.9975
  Constant2 : Constant  Value=0.98
  Constant23 : Constant  Value=0.98
  Constant24 : Constant  Value=0.952
  Constant26 : Constant  Value=0.907
  Constant27 : Constant  Value=0.952
  Constant28 : Constant  Value=0
  Constant29 : Constant  Value=0.907
  Constant4 : Constant  Value=0.9975
  Constant5 : Constant  Value=6.09
  Constant6 : Constant  Value=11.34
  Constant7 : Constant  Value=48.43
  Constant9 : Constant  Value=0.952
  Display : Display
  Gain : Gain  Gain=0
  Gain1 : Gain
  Gain2 : Gain  Gain=0
  Gain3 : Gain
  Gain4 : Gain  Gain=2
  Gain5 : Gain  Gain=6.4
  Gain6 : Gain  Gain=11.75
  Gain7 : Gain  Gain=48.96
  Gain8 : Gain  Gain=2
  GreaterThan{1,12..13,18} (4 alike) : RelationalOperator  Operator=<=  OutDataTypeStr=boolean  RndMeth=Simplest  InputSameDT=off
  GreaterThan16 : RelationalOperator  OutDataTypeStr=boolean  RndMeth=Simplest  InputSameDT=off
  GreaterThan{2,4,6,17,19} (5 alike) : RelationalOperator  Operator=>  OutDataTypeStr=boolean  RndMeth=Simplest  InputSameDT=off
  Multiport Switch : MultiPortSwitch  DataPortOrder=Zero-based contiguous  DataPortForDefault=Additional data port  zeroidx=on  SaturateOnIntegerOverflow=off  InputSameDT=off
  Sum1 : Sum  Inputs=+++
  Sum2 : Sum  Inputs=+-
  Sum3 : Sum  Inputs=+-
  Sum4 : Sum  Inputs=+-
  Sum6 : Sum  Inputs=+++
  Mode : Outport
  Holding Angle : Outport  Port=2
  wires:
  Constant27/1 -> GreaterThan13/2
  Constant24/1 -> GreaterThan19/2
  Constant26/1 -> GreaterThan12/2
  Constant29/1 -> GreaterThan17/2
  GreaterThan17/1 -> AND1/1
  Constant23/1 -> GreaterThan18/2
  Constant28/1 -> GreaterThan16/2
  GreaterThan19/1 -> AND2/1
  GreaterThan12/1 -> AND/2
  GreaterThan16/1 -> AND/1
  GreaterThan18/1 -> AND2/2
  GreaterThan13/1 -> AND1/2
  AND/1 -> Gain/1  "Linear"
  AND1/1 -> Gain1/1  "Mode I"
  AND2/1 -> Gain2/1  "Mode II.I"
  Gain1/1 -> Sum6/2
  Gain/1 -> Sum6/1
  Sum6/1 -> Mode/1
  GreaterThan1/1 -> AND3/2
  AND3/1 -> Gain3/1  "Mode II.II"
  Constant1/1 -> GreaterThan1/2
  Constant2/1 -> GreaterThan2/2
  GreaterThan2/1 -> AND3/1
  Constant4/1 -> GreaterThan4/2
  GreaterThan4/1 -> Gain4/1  "Mode II.III"
  Gain3/1 -> Sum1/2
  Gain4/1 -> Sum1/3
  Gain2/1 -> Sum1/1
  Sum1/1 -> Display/1, Multiport Switch/1
  Gain5/1 -> Sum2/1
  Constant5/1 -> Sum2/2
  Sum2/1 -> Multiport Switch/2
  Sum3/1 -> Multiport Switch/3
  Constant6/1 -> Sum3/2
  Gain6/1 -> Sum3/1
  Gain7/1 -> Sum4/1
  Constant7/1 -> Sum4/2
  Sum4/1 -> Multiport Switch/4
  Multiport Switch/1 -> Holding Angle/1
  M/1 -> GreaterThan16/1, GreaterThan12/1, GreaterThan17/1, GreaterThan13/1, GreaterThan19/1, GreaterThan4/1, Gain7/1, Gain6/1, Gain5/1, GreaterThan1/1, GreaterThan2/1, GreaterThan18/1, GreaterThan6/1
  Gain8/1 -> Sum6/3
  GreaterThan6/1 -> Gain8/1  "Mode II"
  Constant9/1 -> GreaterThan6/2
  Constant/1 -> Multiport Switch/5

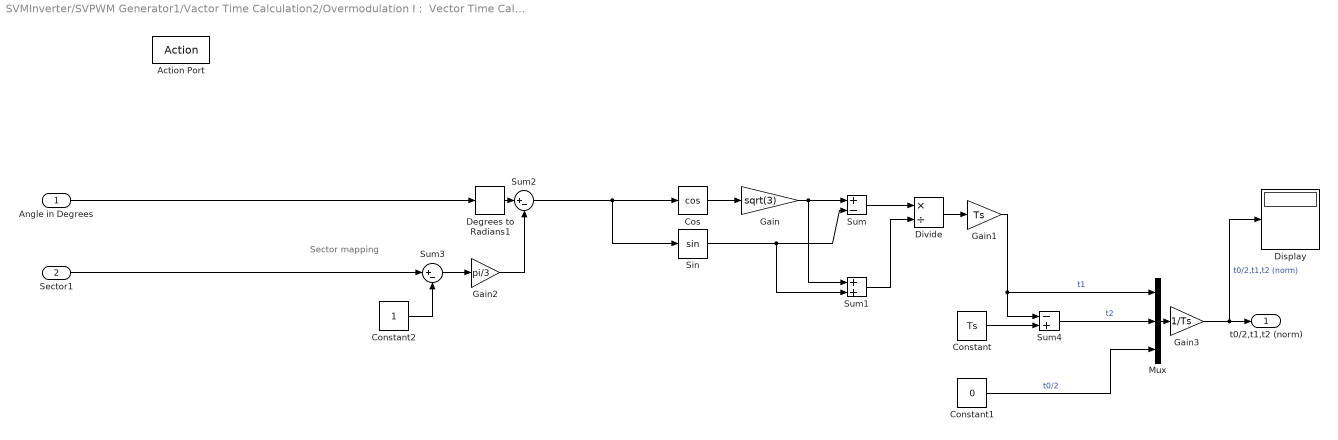
== system SVMInverter/SVPWM Generator1/Vactor Time Calculation2/Overmodulation I :  Vector Time Calculation ==
  note: Sector mapping
  "Angle in Degrees " : Inport
  Sector1 : Inport  Port=2
  Action Port : ActionPort  InitializeStates=reset  ActionPortLabel=case [ 1 ]:
  Constant : Constant  Value=Ts
  Constant1 : Constant  Value=0
  Constant2 : Constant
  Cos : Trigonometry  Operator=cos
  Degrees to Radians1 : simulink_extras/Transformations/Degrees to Radians
  Display : Display
  Divide : Product  Inputs=*/
  Gain : Gain  Gain=sqrt(3)
  Gain1 : Gain  Gain=Ts
  Gain2 : Gain  Gain=pi/3
  Gain3 : Gain  Gain=1/Ts
  Mux : Mux  Inputs=3
  Sin : Trigonometry
  Sum : Sum  Inputs=+-
  Sum1 : Sum
  Sum2 : Sum  Inputs=|+-
  Sum3 : Sum  Inputs=|+-
  Sum4 : Sum  Inputs=-+
  t0/2,t1,t2 (norm) : Outport
  wires:
  Degrees to Radians1/1 -> Sum2/1
  Sector1/1 -> Sum3/1
  Sum3/1 -> Gain2/1
  Constant2/1 -> Sum3/2
  "Angle in Degrees "/1 -> Degrees to Radians1/1
  Gain3/1 -> Display/1, t0/2,t1,t2 (norm)/1  "t0/2,t1,t2 (norm)"
  Gain2/1 -> Sum2/2
  Cos/1 -> Gain/1
  Gain/1 -> Sum1/1, Sum/1
  Sin/1 -> Sum1/2, Sum/2
  Sum/1 -> Divide/1
  Sum1/1 -> Divide/2
  Divide/1 -> Gain1/1
  Constant/1 -> Sum4/2
  Sum4/1 -> Mux/2  "t2"
  Sum2/1 -> Sin/1, Cos/1
  Constant1/1 -> Mux/3  "t0/2"
  Mux/1 -> Gain3/1
  Gain1/1 -> Mux/1, Sum4/1  "t1"

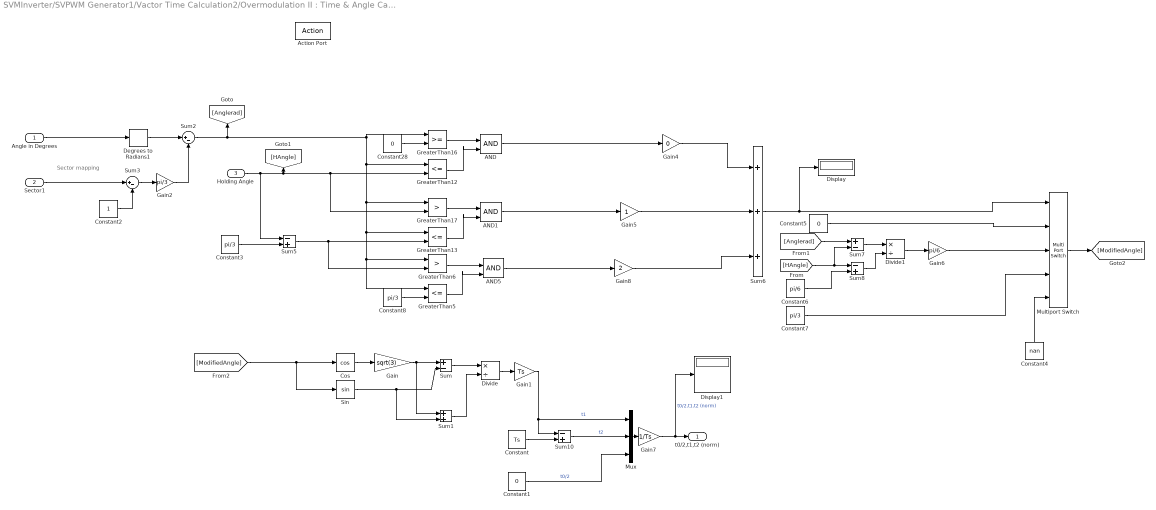
== system SVMInverter/SVPWM Generator1/Vactor Time Calculation2/Overmodulation II : Time & Angle Calculation ==
  note: Sector mapping
  "Angle in Degrees " : Inport
  Sector1 : Inport  Port=2
  Holding Angle : Inport  Port=3
  Action Port : ActionPort  InitializeStates=reset  ActionPortLabel=case [ 2 ]:
  AND : Logic  IconShape=distinctive  AllPortsSameDT=off  OutDataTypeStr=boolean
  AND1 : Logic  IconShape=distinctive  AllPortsSameDT=off  OutDataTypeStr=boolean
  AND5 : Logic  IconShape=distinctive  AllPortsSameDT=off  OutDataTypeStr=boolean
  Constant : Constant  Value=Ts
  Constant1 : Constant  Value=0
  Constant2 : Constant
  Constant28 : Constant  Value=0
  Constant3 : Constant  Value=pi/3
  Constant4 : Constant  Value=nan
  Constant5 : Constant  Value=0
  Constant6 : Constant  Value=pi/6
  Constant7 : Constant  Value=pi/3
  Constant8 : Constant  Value=pi/3
  Cos : Trigonometry  Operator=cos
  Degrees to Radians1 : simulink_extras/Transformations/Degrees to Radians
  Display : Display
  Display1 : Display
  Divide : Product  Inputs=*/
  Divide1 : Product  Inputs=*/
  Gain : Gain  Gain=sqrt(3)
  Gain1 : Gain  Gain=Ts
  Gain2 : Gain  Gain=pi/3
  Gain4 : Gain  Gain=0
  Gain5 : Gain
  Gain6 : Gain  Gain=pi/6
  Gain7 : Gain  Gain=1/Ts
  Gain8 : Gain  Gain=2
  GreaterThan12 : RelationalOperator  Operator=<=  OutDataTypeStr=boolean  RndMeth=Simplest  InputSameDT=off
  GreaterThan13 : RelationalOperator  Operator=<=  OutDataTypeStr=boolean  RndMeth=Simplest  InputSameDT=off
  GreaterThan16 : RelationalOperator  OutDataTypeStr=boolean  RndMeth=Simplest  InputSameDT=off
  GreaterThan17 : RelationalOperator  Operator=>  OutDataTypeStr=boolean  RndMeth=Simplest  InputSameDT=off
  GreaterThan5 : RelationalOperator  Operator=<=  OutDataTypeStr=boolean  RndMeth=Simplest  InputSameDT=off
  GreaterThan6 : RelationalOperator  Operator=>  OutDataTypeStr=boolean  RndMeth=Simplest  InputSameDT=off
  Multiport Switch : MultiPortSwitch  DataPortOrder=Zero-based contiguous  DataPortForDefault=Additional data port  zeroidx=on  SaturateOnIntegerOverflow=off  InputSameDT=off
  Mux : Mux  Inputs=3
  Sin : Trigonometry
  Sum : Sum  Inputs=+-
  Sum1 : Sum
  Sum10 : Sum  Inputs=-+
  Sum2 : Sum  Inputs=|+-
  Sum3 : Sum  Inputs=|+-
  Sum5 : Sum  Inputs=-+
  Sum6 : Sum  Inputs=+++
  Sum7 : Sum  Inputs=+-
  Sum8 : Sum  Inputs=-+
  t0/2,t1,t2 (norm) : Outport
  wires:
  Sum5/1 -> GreaterThan6/2, GreaterThan13/2
  GreaterThan6/1 -> AND5/1
  GreaterThan16/1 -> AND/1
  Gain8/1 -> Sum6/3
  GreaterThan5/1 -> AND5/2
  Gain5/1 -> Sum6/2
  AND5/1 -> Gain8/1
  Sum6/1 -> Display/1, Multiport Switch/1
  AND/1 -> Gain4/1
  GreaterThan17/1 -> AND1/1
  AND1/1 -> Gain5/1
  Constant28/1 -> GreaterThan16/2
  GreaterThan13/1 -> AND1/2
  GreaterThan12/1 -> AND/2
  Gain4/1 -> Sum6/1
  Holding Angle/1 -> [HAngle], GreaterThan17/2, GreaterThan12/2, Sum5/1
  Constant8/1 -> GreaterThan5/2
  Constant3/1 -> Sum5/2
  Constant4/1 -> Multiport Switch/5
  Constant5/1 -> Multiport Switch/2
  Gain6/1 -> Multiport Switch/3
  [Anglerad] -> Sum7/1
  [HAngle] -> Sum8/1, Sum7/2
  Constant6/1 -> Sum8/2
  Sum7/1 -> Divide1/1
  Sum8/1 -> Divide1/2
  Divide1/1 -> Gain6/1
  Constant7/1 -> Multiport Switch/4
  Multiport Switch/1 -> [ModifiedAngle]
  Sum2/1 -> GreaterThan16/1, GreaterThan12/1, GreaterThan17/1, GreaterThan13/1, GreaterThan5/1, GreaterThan6/1, [Anglerad]
  Sum3/1 -> Gain2/1
  Gain2/1 -> Sum2/2
  Sector1/1 -> Sum3/1
  Constant2/1 -> Sum3/2
  Degrees to Radians1/1 -> Sum2/1
  "Angle in Degrees "/1 -> Degrees to Radians1/1
  Gain1/1 -> Mux/1, Sum10/1  "t1"
  Mux/1 -> Gain7/1
  Sum1/1 -> Divide/2
  Constant/1 -> Sum10/2
  Sum10/1 -> Mux/2  "t2"
  Gain7/1 -> Display1/1, t0/2,t1,t2 (norm)/1  "t0/2,t1,t2 (norm)"
  Divide/1 -> Gain1/1
  Constant1/1 -> Mux/3  "t0/2"
  Sum/1 -> Divide/1
  Gain/1 -> Sum1/1, Sum/1
  [ModifiedAngle] -> Sin/1, Cos/1
  Sin/1 -> Sum1/2, Sum/2
  Cos/1 -> Gain/1

== matlab function SVMInverter/Rotation Matrix/MATLAB Function1 ==
  data: x input; AB output; th input
function AB = Rot(x,th)

P=[ cos(th) -sin(th);
     sin(th) cos(th)];

AB=P*x;

== matlab function SVMInverter/SVPWM Generator1/Off time per sector calculator/Off time per sector calculator ==
  data: toff input; Tmat output; sector input
function Tmat = Sectortime(toff,sector)


switch sector
    case 1
        Tmat=toff(1:3);
    case 2
        Tmat=toff(4:6);
    case 3
        Tmat=toff(7:9);
    case 4
        Tmat=toff(10:12);
    case 5
        Tmat=toff(13:15);
    case 6
        Tmat=toff(16:18);
    otherwise
        Tmat=[inf;inf;inf];
end

== matlab function SVMInverter/ClarkT/MATLAB Function1 ==
  data: x input; alpha output; beta output
function [alpha,beta] = Clark(x)
P=(2/3)*[ cos(0) cos(0-2*pi/3) cos(0+2*pi/3);
         -sin(0) -sin(0-2*pi/3) -sin(0+2*pi/3)  ];
prod=P*x;
alpha=prod(1);
beta=prod(2);

== matlab function SVMInverter/ParkT/MATLAB Function1 ==
  data: x input; dq output; th input
function dq = Park(x,th)
% vd=(2/3)*(u1*cos(th)+u2*cos(th-2*pi/3)+u3*cos(th+2*pi/3));
% vq=(2/3)*(-u1*sin(th)-u2*sin(th-2*pi/3)-u3*sin(th+2*pi/3));
P=(2/3)*[ cos(th) cos(th-2*pi/3) cos(th+2*pi/3);
         -sin(th) -sin(th-2*pi/3) -sin(th+2*pi/3)  ];
dq=P*x;
% xd=prod(1);
% xq=prod(2);

== matlab function SVMInverter/SVPWM Generator/Off time per sector calculator/Off time per sector calculator ==
  data: toff input; Tmat output; sector input
function Tmat = Sectortime(toff,sector)


switch sector
    case 1
        Tmat=toff(1:3);
    case 2
        Tmat=toff(4:6);
    case 3
        Tmat=toff(7:9);
    case 4
        Tmat=toff(10:12);
    case 5
        Tmat=toff(13:15);
    case 6
        Tmat=toff(16:18);
    otherwise
        Tmat=[inf;inf;inf];
end
